simulink model "Model_TranslationEngine64"  (R2022b)
settings: Solver=FixedStepDiscrete  StartTime=0.0  StopTime=5  RelTol=1e-3  EnableMultiTasking=on
InitFcn:
  | % Initialize model
  | ModelSettings=BTConfig.GetModelSettings();
  | 
  | ModelSettings.Validate();
  | 
  | ModelInit;
  | 
  | 
  | % load library data
  | GainLibrary_data;
  | % Load saved values from partition process
  | CapturedConstMask.LoadMapFromFile(bdroot)
StartFcn:
  | % make sure all the simulated RTC requests are found
  | %RTC_SIM_OBJ.ValidateREQs();
undefined symbols (not defined in the file or in its folder): AA, BPLP, Column, NumHFRefBPF, NumHFRefLPF, NumMusicChannels, Row, VolumeMuteConfig
libraries: TuneVar x925, TOP x490, FeaturePath x111, CapturedConstLib x52
(part 34 of 34)

== matlab function Model_TranslationEngine64/ModelPreAmp/DecRate/Medusa5H1/MedusaHoligram/Medusa5H1 Part 3/On/Expand Tail Components/Tail Component EQ/InnerLink/PoolIirTunableWithReset/Translation ==
  data: RawSOS input; NumStages input; PoolNumStages output; PoolCoeffs output; MaxNumStages parameter; VariantUint8 parameter; NumChannels input
  events: trigger input FUNCTION_CALL_EVENT
function [PoolNumStages, PoolCoeffs] = pooliirTranslation(RawSOS, NumStages, MaxNumStages, VariantUint8,  NumChannels)
%#codegen

% Translation from raw SOS for pool SOS

% Some build time sanity size checking before calling the translation
if numel(NumStages.Value) ~= NumChannels
    error('Size of num stages has to match number of input channels')
end

if RawSOS.Size(2) ~= 6
    error ('Coefficient pool matrix must have 6 columns')
end

[PoolNumStages, PoolCoeffs] = poolIirTranslation(RawSOS, NumStages, MaxNumStages, VariantUint8);

% VariantStr = char(VariantUint8);
% switch (VariantStr)
%     case {"Generic","SharcPlusCore"}
%         % These variants order biquad coefficients in a compacted form
%         [PoolNumStages, PoolCoeffs] = pooliirTranslationFcn(RawSOS, NumStages, MaxNumStages);
%     case {"SharcPlusAccelGul","SharcPlusAccelGxp"}
%         % These variants order biquad coefficients for the ADI accelerator
%         [PoolNumStages, PoolCoeffs] = pooliirAccelTranslationFcn(RawSOS, NumStages, MaxNumStages);
%     case{"Hexagon"}
%         % Hexagon specific order for biquad coefficients 
%         [PoolNumStages, PoolCoeffs] = PoolIirHexagonTranslationFcn(RawSOS, NumStages, MaxNumStages);
%     case{"ArmNeonV7V8"}
%         [PoolNumStages, PoolCoeffs] = PoolIirArmNeonV7V8TranslationFcn(RawSOS, NumStages, MaxNumStages);
%     otherwise
%         % This is a build-time error, not a translation error. The
%         % selected build-time variant is not supported for translation
%         error('Invalid implementation type: [%s]', VariantStr);
% end

end

== matlab function Model_TranslationEngine64/NEAR/Near1p1/VolumeMute/VolMuteCh1/Ann1NonEntVncApplied/nonentVNCApplied_subsystem/TuneTOP/Translation ==
  data: Num output; tau input; Fs input; L input; Den output
  events: trigger input FUNCTION_CALL_EVENT
function [Num, Den]  = fcn(tau, Fs, L)

f0 = 1/tau.Value;   % Approximation of cutoff freq from lpf filter time constant

fs_lpf = Fs/L;        % lpf filtter sample rate

% [Num, Den]= butter(1,2*f0/fs_lpf);  % butter() doesn't work with dynamic parameters
[Num, Den] = firstOrderButter(fs_lpf,f0);  % Calculation of lpf filter coefficients

== matlab function Model_TranslationEngine64/ModelPreAmp/DecRate/Medusa5H1/MedusaHoligram/Medusa5H1 Part 2/SPUM Decay Estimate/Decay Estimate/Trivial Translation ==
  data: PSDSmoothFactor output; PSDSmoothCutoff input; FrameRate input
  events: trigger input FUNCTION_CALL_EVENT
function PSDSmoothFactor  = fcn(PSDSmoothCutoff, FrameRate)
% Cutoff is the inverse of time constant in Hz. So this function
% basically converts reciprocal of time constant to first order iir
% filter coefficient.
% Reference: https://bosecorp.sharepoint.com/sites/ASD3/DSPTeam/Shared%20Documents/DSP_Topics/Comparison%20of%20time%20constant%20conversion%20methods.docx
wn = 2 * pi * PSDSmoothCutoff.Value / FrameRate;
PSDSmoothFactor = (1 - sin(wn)) ./ cos(wn);
end

== matlab function Model_TranslationEngine64/ModelPreAmp/DecRate/Medusa5H1/MedusaHoligram/Medusa5H1 Part 2/SPUM Decay Estimate/Decay Estimate/Trivial Translation1 ==
  data: DecaySmoothFactor output; DecaySmoothCutoff input; FrameRate input
  events: trigger input FUNCTION_CALL_EVENT
function DecaySmoothFactor  = fcn(DecaySmoothCutoff, FrameRate)
% Cutoff is the inverse of time constant in Hz. So this function
% basically converts reciprocal of time constant to first order iir
% filter coefficient.
% Reference: https://bosecorp.sharepoint.com/sites/ASD3/DSPTeam/Shared%20Documents/DSP_Topics/Comparison%20of%20time%20constant%20conversion%20methods.docx
wn = 2 * pi * DecaySmoothCutoff.Value / FrameRate;
DecaySmoothFactor = (1 - sin(wn)) ./ cos(wn);
end

== matlab function Model_TranslationEngine64/ModelPreAmp/DecRate/Medusa5H1/MedusaHoligram/Medusa5H1 Part 2/SPUM Decay Estimate/Decay Estimate/Trivial Translation2 ==
  data: FastAttack output; FastAttackCutoff input; SlowAttackCutoff input; FrameRate input; SlowAttack output
  events: trigger input FUNCTION_CALL_EVENT
function [FastAttack, SlowAttack] = fcn(FastAttackCutoff, SlowAttackCutoff, FrameRate)
% Cutoff is the inverse of time constant in Hz. So this function
% basically converts reciprocal of time constant to first order iir
% filter coefficient.
% Reference: https://bosecorp.sharepoint.com/sites/ASD3/DSPTeam/Shared%20Documents/DSP_Topics/Comparison%20of%20time%20constant%20conversion%20methods.docx
if FastAttackCutoff.Value >= SlowAttackCutoff.Value
    wn = 2 * pi * FastAttackCutoff.Value / FrameRate;
    FastAttack = 1 - (1 - sin(wn)) ./ cos(wn);
    wn = 2 * pi * SlowAttackCutoff.Value / FrameRate;
    SlowAttack = 1 - (1 - sin(wn)) ./ cos(wn);
else
    TranslateError('Cutoff frequency of single pole averager for '...
        ,'decay should be less than or equal to that for attack');
    FastAttack = 0;
    SlowAttack = 0;
end

== matlab function Model_TranslationEngine64/ModelPreAmp/DecRate/Medusa5H1/MedusaHoligram/Medusa5H1 Part 2/SPUM Decay Estimate/Decay Estimate/Trivial Translation3 ==
  data: StepIncrement output; StepSize input; FrameRate input; StepDecrement output
  events: trigger input FUNCTION_CALL_EVENT
function [StepIncrement, StepDecrement] = fcn(StepSize, FrameRate)

if StepSize.Value >= 0
    StepIncrement = StepSize.Value/FrameRate;
    StepDecrement = -StepSize.Value/FrameRate;
else
    TranslateError('Step size for slewing should be greater than or equal to zero.');
    StepIncrement = 0;
    StepDecrement = 0;
end

== matlab function Model_TranslationEngine64/ModelPreAmp/DecRate/Medusa5H1/MedusaHoligram/Medusa5H1 Part 2/SPUM Decay Estimate/Decay Estimate/Trivial Translation4 ==
  data: directPathSec input; FrameRate input; DirectPathFramesFs output
  events: trigger input FUNCTION_CALL_EVENT
function DirectPathFramesFs  = fcn(directPathSec, FrameRate)

% Convert delay in seconds to number of full-rate frames
DirectPathFramesFs = round(directPathSec.Value*FrameRate);

end

== matlab function Model_TranslationEngine64/ModelPreAmp/DecRate/Medusa5H1/MedusaHoligram/Medusa5H1 Part 2/Full-Rate FDP/Fdp/FreqDomainProcessing/CalculateAndApplyCoefficients/FullRate/Calculate coefficients/StretchParams/Trivial Translation ==
  data: XpMax output; XpMaxIn input; LokRokMaxScaleFactor output; XpMinIn input; XpMin output; deciXpMaxIn input
  events: trigger input FUNCTION_CALL_EVENT
function [XpMax, LokRokMaxScaleFactor,  XpMin] = fcn(XpMaxIn, XpMinIn, deciXpMaxIn)

XpMax = XpMaxIn.Value;
XpMin = XpMinIn.Value;

if (XpMin < 0) || (XpMin >= 1)
    TranslateError('XpMin must be no less than 0.0, and must be less than 1.0');
end

if (XpMax < 0) || (XpMax >= 1)
    TranslateError('XpMax must be no less than 0.0, and must be less than 1.0');
end

if (XpMax < XpMin)
    TranslateError('XpMin cannot exceed XpMax');
end

% Do not need to check for translation error as this is already done in
% Decimated Rate block.
deciXpMax = deciXpMaxIn.Value; 

% NOTE: The Xp used for detect is the decimated rate Xp while the Xp
% used for the XpMax (in the dynamically created Xp) is the treble Xp.
% All parameters are also treble-specific (different from decimated rate).
% This means the LokRokMaxScaleFactor for treble stretching is calculated
% using the decimated rate XpMax.
if (deciXpMax == 1)
    LokRokMaxScaleFactor = 0;
else
    LokRokMaxScaleFactor = 0.5 * deciXpMax / (1 - deciXpMax);
end

end

== matlab function Model_TranslationEngine64/ModelPreAmp/DecRate/Medusa5H1/MedusaHoligram/Medusa5H1 Part 2/Full-Rate FDP/Fdp/FreqDomainProcessing/CalculateAndApplyCoefficients/FullRate/Calculate coefficients/StretchParams/Trivial Translation3 ==
  data: ESDUpperbounddBIn input; ESDUpperbounddB output; ESDLowerbounddB output; ESDLowerbounddBIn input; ESDStepSize output
  events: trigger input FUNCTION_CALL_EVENT
function [ESDUpperbounddB, ESDLowerbounddB, ESDStepSize]  = ...
                fcn(ESDUpperbounddBIn, ESDLowerbounddBIn)
            
if (ESDUpperbounddBIn.Value >= ESDLowerbounddBIn.Value)
    ESDUpperbounddB = ESDUpperbounddBIn.Value;
    ESDLowerbounddB = ESDLowerbounddBIn.Value;
else    
    TranslateError('Lower threshold for ESD cannot exceed upper threshold for ESD');
    ESDUpperbounddB = 0;
    ESDLowerbounddB = 0;
end

if (ESDUpperbounddBIn.Value == ESDLowerbounddBIn.Value)
    ESDStepSize = 0;
else
    ESDStepSize = 1/abs(ESDUpperbounddBIn.Value - ESDLowerbounddBIn.Value);
end

end

== matlab function Model_TranslationEngine64/ModelPreAmp/DecRate/Medusa5H1/MedusaHoligram/Medusa5H1 Part 4/On/DR Mix Matrix with Hybrid Holigram EQ/IIR/PoolIirTunableWithReset/Translation ==
  data: RawSOS input; NumStages input; PoolNumStages output; PoolCoeffs output; MaxNumStages parameter; VariantUint8 parameter; NumChannels input
  events: trigger input FUNCTION_CALL_EVENT
function [PoolNumStages, PoolCoeffs] = pooliirTranslation(RawSOS, NumStages, MaxNumStages, VariantUint8,  NumChannels)
%#codegen

% Translation from raw SOS for pool SOS

% Some build time sanity size checking before calling the translation
if numel(NumStages.Value) ~= NumChannels
    error('Size of num stages has to match number of input channels')
end

if RawSOS.Size(2) ~= 6
    error ('Coefficient pool matrix must have 6 columns')
end

[PoolNumStages, PoolCoeffs] = poolIirTranslation(RawSOS, NumStages, MaxNumStages, VariantUint8);

% VariantStr = char(VariantUint8);
% switch (VariantStr)
%     case {"Generic","SharcPlusCore"}
%         % These variants order biquad coefficients in a compacted form
%         [PoolNumStages, PoolCoeffs] = pooliirTranslationFcn(RawSOS, NumStages, MaxNumStages);
%     case {"SharcPlusAccelGul","SharcPlusAccelGxp"}
%         % These variants order biquad coefficients for the ADI accelerator
%         [PoolNumStages, PoolCoeffs] = pooliirAccelTranslationFcn(RawSOS, NumStages, MaxNumStages);
%     case{"Hexagon"}
%         % Hexagon specific order for biquad coefficients 
%         [PoolNumStages, PoolCoeffs] = PoolIirHexagonTranslationFcn(RawSOS, NumStages, MaxNumStages);
%     case{"ArmNeonV7V8"}
%         [PoolNumStages, PoolCoeffs] = PoolIirArmNeonV7V8TranslationFcn(RawSOS, NumStages, MaxNumStages);
%     otherwise
%         % This is a build-time error, not a translation error. The
%         % selected build-time variant is not supported for translation
%         error('Invalid implementation type: [%s]', VariantStr);
% end

end

== matlab function Model_TranslationEngine64/ModelPreAmp/DecRate/Medusa5H1/MedusaHoligram/Medusa5H1 Part 3/On/VLS Gains Computation/VLS Gains Drv/Fade Tuning/Backward Downmix Max/Trivial Translation ==
  data: TOP output; BackwardDownmixMax input
  events: trigger input FUNCTION_CALL_EVENT
function TOP  = fcn(BackwardDownmixMax)
%#codegen
% Checks if the parameter satisfies dimensionality requirements
if(numel(BackwardDownmixMax.Value) ~= 1)
   TranslateError('The parameter ''medusa_backward_downmix_max'' must be single dimensional.'); 
end

% Checks if the parameter value follows bound requirements
if((BackwardDownmixMax.Value < 0) || (BackwardDownmixMax.Value > 1))
   TranslateError('The value of ''medusa_backward_downmix_max'' must be between 0 and 1.'); 
end

TOP = BackwardDownmixMax.Value;

end

== matlab function Model_TranslationEngine64/ModelPreAmp/DecRate/Medusa5H1/MedusaHoligram/Medusa5H1 Part 2/Decimated-Rate FDP/Fdp/FreqDomainProcessing/Reverb Extractions/Trivial Translation1 ==
  data: FastPsdSmoothFactor output; FastPsdSmoothCutoff input; SlowPsdSmoothFactor output; SlowPsdSmoothCutoff input; FrameRate input
  events: trigger input FUNCTION_CALL_EVENT
function [FastPsdSmoothFactor, SlowPsdSmoothFactor]  = fcn(FastPsdSmoothCutoff, SlowPsdSmoothCutoff, FrameRate)
% Cutoff is the inverse of time constant in Hz. So this function
% basically converts reciprocal of time constant to first order iir
% filter coefficient.
% Reference: https://bosecorp.sharepoint.com/sites/ASD3/DSPTeam/Shared%20Documents/DSP_Topics/Comparison%20of%20time%20constant%20conversion%20methods.docx

if FastPsdSmoothCutoff.Value >= SlowPsdSmoothCutoff.Value
    wn = 2 * pi * FastPsdSmoothCutoff.Value / FrameRate;
    FastPsdSmoothFactor = (1 - sin(wn)) ./ cos(wn);
    wn = 2 * pi * SlowPsdSmoothCutoff.Value / FrameRate;
    SlowPsdSmoothFactor = (1 - sin(wn)) ./ cos(wn);
else
    TranslateError('Cutoff frequency of single pole averager for smoothing'... 
       ,'fast PSD should be less than or equal to that for smoothing slow PSD.');
    FastPsdSmoothFactor = 0;
    SlowPsdSmoothFactor = 0;
end

== matlab function Model_TranslationEngine64/NEAR/Near1p1/NearBandSplit/HighpassFilter/Translation ==
  data: LRHighPassNumStages output; LRHighPassCoeffs output; crossOverFrequency input; order input; sampleRate input; numChannels input
  events: trigger input FUNCTION_CALL_EVENT
function [LRHighPassNumStages, LRHighPassCoeffs]  = fcn(crossOverFrequency, order, sampleRate, numChannels)
%#codegen
MAX_HPF_ORDER = 10;
MAX_NUM_CHANNELS = 4;
IIR_HIGHPASS = 1;

% Linkwitz-Riley Filters can be construed as the cascade of
% two Butterworth Filters of half the order at the same frequency.
filterOrder = order.Value;
butterOrder = floor((filterOrder+1)/2);
normFrequency = crossOverFrequency.Value/(sampleRate/2);

% High-pass Filters
[halfZ, halfP, halfK] = CalcButterworth(butterOrder,normFrequency,IIR_HIGHPASS);
fullZ = [halfZ halfZ];                         % zeros
fullP = [halfP halfP];                         % poles
fullK = halfK*halfK;                           % gain
sosHighPass = zp2sos(fullZ,fullP,fullK);

% Generate Linkwitz-Riley Pair Coefficients
maxFilterOrder = MAX_HPF_ORDER;
maxNumChannels = MAX_NUM_CHANNELS;
numStages = uint32(size(sosHighPass, 1) * ones(1, maxNumChannels));
maxNumStages = maxFilterOrder * maxNumChannels;

LRHighPassNumStages = uint32(zeros(maxNumChannels,1));
LRHighPassCoeffs = single(zeros((maxNumStages * 4 + maxNumChannels),1));

rawSOSHighPass = repmat(sosHighPass, 4, 1);
[LRHighPassNumStages, LRHighPassCoeffs] = pooliirTranslation(rawSOSHighPass, numStages, maxNumStages, numChannels, maxNumChannels);

end

function [PoolNumStages, PoolCoeffs] = pooliirTranslation(rawSOS, numStages, maxNumStages, numChannels, maxNumChannels)

RawSOS = rawSOS;
NumStages = uint32(numStages);
NumChannels = numChannels;

MaxNumStages = maxNumStages; 
PoolNumStages = uint32(zeros(maxNumChannels,1));
PoolCoeffs = single(zeros(MaxNumStages * 4 + maxNumChannels,1));
ChannelCoeffs = zeros(MaxNumStages * 4 + 1,1);
ChannelSOS = single(zeros(MaxNumStages, 6));
SOSIndex = uint32(0);


for i = 1:NumChannels
    
    ChannelNumStages = NumStages(i);   % Size of current SOS
    assert(ChannelNumStages <= MaxNumStages);
    
    if (ChannelNumStages == 0)
        continue;
    end
    
    ChannelSOS(1:ChannelNumStages,:) = RawSOS(SOSIndex+(1:ChannelNumStages),:);
    SOSIndex = SOSIndex + ChannelNumStages;

    if size(ChannelSOS,2) ~= 6
        TranslateError('SOS matrix must have 6 columns');
    end
    % decompose SOS
   
    ts = 1:4:4*ChannelNumStages;
    ChannelCoeffs(1,1) = prod(ChannelSOS(1:ChannelNumStages,1));        % b0
	
	% Error out for poorly-formed sos coeffs
	if ((ChannelCoeffs(1,1) == 0) && (ChannelNumStages > 1))
		TranslateError('Poorly-formed SOS: zero b0 for multi-stage results in a zero EQ.');
	end
    
    % the remaining coeffs are compacted forms of the biquads
    ChannelCoeffs(1+ts,1) = ChannelSOS(1:ChannelNumStages,6);           % a2
    ChannelCoeffs(2+ts,1) = ChannelSOS(1:ChannelNumStages,5);           % a1
    if( any(ChannelSOS(1:ChannelNumStages,1) == 0 ))
    ChannelCoeffs(3+ts,1) = 0;                 % b2/b0
    ChannelCoeffs(4+ts,1) = 0;                 % b1/b0
    else
    ChannelCoeffs(3+ts,1) = ...
        ChannelSOS(1:ChannelNumStages,3)./ ...
        ChannelSOS(1:ChannelNumStages,1);  % b2/b0
    ChannelCoeffs(4+ts,1) = ...
        ChannelSOS(1:ChannelNumStages,2)./ ...
        ChannelSOS(1:ChannelNumStages,1);  % b1/b0
    end
    
    % length of Cuurent Channel Coeffs
    
    ChannelCoeffsLength = 1+4*ChannelNumStages;
    
    % Offset into coefficient array for the current channel
    offset = uint32((i-1)+4*sum(PoolNumStages(1:i-1)));
    
    % Verify that the SOS does not violate the maximum number of stages
    % allocated for the pool
    PoolNumStages(i) = int32(ChannelNumStages);
    if sum(PoolNumStages) > MaxNumStages
        TranslateError('Too many second order sections');
    end

    % Store the coefficients
    PoolCoeffs(offset+(1:ChannelCoeffsLength)) = single(ChannelCoeffs(1:ChannelCoeffsLength));   
end
end

function [z,p,k] = CalcButterworth(order,frequency,filterType)
MAX_HPF_ORDER = 10;
IIR_HIGHPASS = 1;

    if order > MAX_HPF_ORDER
       order = MAX_HPF_ORDER;
    end
            
    % zeros first
    z = zeros(1,order);
    if filterType == IIR_HIGHPASS
        z(1:order) = ones(1,min(order,MAX_HPF_ORDER));
    elseif filterType == IIR_LOWPASS
        z(1:order) = -1*ones(1,min(order,MAX_HPF_ORDER));
    else
        TranslateError('Filter Type must be high or low');
    end

    p = complex(zeros(1,MAX_HPF_ORDER));
    for n = 1:order
        if n == (order+1)/2 
            sp = -pi*frequency;
        else
            sp_real = pi*frequency*cos(((2*n+order-1)*pi)/(2*order));
            sp_imag = pi*frequency*sin(((2*n+order-1)*pi)/(2*order));
            sp = sp_real + 1i*sp_imag;
        end

        p(n) = (1+sp/2)/(1-sp/2);
    end

    z = z(1:order);
    p = p(1:order);

    if filterType == IIR_HIGHPASS
        k = real(prod((1+p(1:order))/2));
    else 
        k = real(prod((1-p(1:order))/2));
    end
end

% The zp2sos Function stated below supports code generation! 
% Most of the code is scripted refering to the Matlab's zp2sos.m and
% https://searchcode.com/codesearch/view/9505959/ 
% Integration of two codes was majorily required due to cplxreal function 
% which is no more supported in Matlab Scripts. 
function [sos,g] = zp2sos(z,p,g)
    if nargin < 3
        g = 1; 
    end
    if nargin < 2
        p = []; 
    end

    % Sort the numbers z into complex-conjugate-valued and real-valued elements.
    % The positive imaginary complex numbers of each complex conjugate pair 
    % are returned in zc and the real numbers are returned in zr.

    % pair up the conjugate poles and zeros using cplxpair
    z = cplxpair(z);
    p = cplxpair(p);

    % Get the number of poles and zeros
    lz = length(z);
    lp = length(p);

    ind = find(abs(imag(p)) > 0);
    p_conj = p(ind);   % poles that have conjugate pairs

    coder.varsize('ind_complement');
    B = p_conj(imag(p_conj) >= 0);
    ind_complement = 1:lp;
    if ~isempty(ind)
        ind_complement(ind) = [];
    end
    p_real = p(ind_complement);    % poles that are real

    % break up conjugate pairs and real zeros
    ind = find(abs(imag(z)) > 0);
    z_conj = z(ind);   % zeros that have conjugate pairs
    C = z_conj(imag(z_conj) >= 0);
    ind_complement = 1:lz;
    if ~isempty(ind)
       ind_complement(ind) = [];
    end
    z_real = z(ind_complement);

    zr = z_real; % zeroes that are real
    pr = p_real ;% poles that are real
    pc = B; % positive conjugate poles
    zc = C ; % positive conjugate zeros

    % zc,zr,pc,pr found

    nzc = length(zc);
    npc = length(pc);

    nzr = length(zr);
    npr = length(pr);

    % Pair up real zeros:
    if nzr
        if mod(nzr,2)==1
            zr_temp = [zr;0]; 
            nzr = nzr+1; 
        else
            zr_temp = zr;
        end
        nzrsec = nzr/2;
        zrms = real(-zr_temp(1:2:nzr-1) - zr_temp(2:2:nzr));
        zrp = real(zr_temp(1:2:nzr-1) .* zr_temp(2:2:nzr));
    else
        nzrsec = 0;
        zrms = 0; 
        zrp = 0;
    end

    % Pair up real poles:
    if npr
        if mod(npr,2) == 1
            pr_temp = [pr;0]; 
            npr = npr+1; 
        else
            pr_temp = pr;
        end
        nprsec = npr/2;
        prms = real(-pr_temp(1:2:npr-1) - pr_temp(2:2:npr));
        prp = real(pr_temp(1:2:npr-1) .* pr_temp(2:2:npr));
    else
        nprsec = 0;
        prp = 0;
        prms = 0;
    end

    nsecs = max(ceil(lz/2), ceil(lp/2));

    % Convert complex zeros and poles to real 2nd-order section form:
    zcm2r = -2*real(zc);
    zca2 = abs(zc) .^ 2;
    pcm2r = -2 * real(pc);
    pca2 = abs(pc) .^ 2;

    sos = zeros(nsecs, 6);
    sos(:,1) = ones(nsecs, 1); % all 2nd-order polynomials are monic
    sos(end,1) = g*sos(end, 1);
    sos(:,4) = ones(nsecs, 1); 

    nzrl = nzc + nzrsec; % index of last real zero section
    nprl = npc + nprsec; % index of last real pole section

    for i = 1:nsecs

        if i <= nzc % lay down a complex zero pair:
            sos(i,2:3) = [zcm2r(i) zca2(i)];
            sos(end,2:3) = g*sos(end,2:3);
        elseif i <= nzrl % lay down a pair of real zeros:
            sos(i,2:3) = [zrms(i-nzc) zrp(i-nzc)];
            sos(end,2:3) = g*sos(end,2:3);
        end  

        if i <= npc % lay down a complex pole pair:
            sos(i,5:6) = [pcm2r(i) pca2(i)];
        elseif i <= nprl % lay down a pair of real poles:
            sos(i,5:6) = [prms(i-npc) prp(i-npc)];
        end  
    end        
end

== matlab function Model_TranslationEngine64/ModelPreAmp/DecRate/Medusa5H1/MedusaHoligram/Medusa5H1 Part 2/Decimated-Rate FDP/Fdp/FreqDomainProcessing/Reverb Extractions/Trivial Translation3 ==
  data: DirectPathDec output; DirectPathSec input; FrameRate input; FrameSize input
  events: trigger input FUNCTION_CALL_EVENT
function DirectPathDec  = fcn(DirectPathSec, FrameRate, FrameSize)

DirectPathDec = round(DirectPathSec.Value*FrameRate)*FrameSize;

end

== matlab function Model_TranslationEngine64/ModelPreAmp/DecRate/Medusa5H1/MedusaHoligram/Medusa5H1 Part 2/Decimated-Rate FDP/Fdp/FreqDomainProcessing/Reverb Extractions/Trivial Translation4 ==
  data: LsSmoothFactor output; LsSmoothCutoff input; FrameRate input
  events: trigger input FUNCTION_CALL_EVENT
function LsSmoothFactor  = fcn(LsSmoothCutoff, FrameRate)

% Cutoff is the inverse of time constant in Hz. So this function
% basically converts reciprocal of time constant to first order iir
% filter coefficient.
% Reference: https://bosecorp.sharepoint.com/sites/ASD3/DSPTeam/Shared%20Documents/DSP_Topics/Comparison%20of%20time%20constant%20conversion%20methods.docx
wn = 2 * pi * LsSmoothCutoff.Value / FrameRate;
LsSmoothFactor = (1 - sin(wn)) ./ cos(wn);

end

== matlab function Model_TranslationEngine64/ModelPreAmp/DecRate/Medusa5H1/MedusaHoligram/Medusa5H1 Part 3/On/VLS Gains Computation/VLS Gains Drv/Fade Tuning/Backward Downmix Threshold/Trivial Translation ==
  data: TOP output; BackwardDownmixThreshold input
  events: trigger input FUNCTION_CALL_EVENT
function TOP  = fcn(BackwardDownmixThreshold)
%#codegen
% Checks if the parameter satisfies dimensionality requirements
if(numel(BackwardDownmixThreshold.Value) ~= 1)
   TranslateError('The parameter ''medusa_backward_downmix_threshold'' must be single dimensional.'); 
end

% Checks if the parameter value follows bound requirements
if((BackwardDownmixThreshold.Value < 0) || (BackwardDownmixThreshold.Value > 1))
   TranslateError('The value of ''medusa_backward_downmix_threshold'' must be between 0 and 1.'); 
end

TOP = BackwardDownmixThreshold.Value;

end

== matlab function Model_TranslationEngine64/ModelPreAmp/DecRate/Medusa5H1/MedusaHoligram/Medusa5H1 Part 3/On/VLS Gains Computation/VLS Gains Drv/Fade Tuning/Downmix Weights/Trivial Translation ==
  data: TOP output; downmix_wts input; configStruct parameter
  events: trigger input FUNCTION_CALL_EVENT
function TOP  = fcn(downmix_wts, configStruct)
%#codegen

% Checks if the parameter satisfies dimensionality requirements
if(downmix_wts.Size(1) ~= configStruct.numGains)
    TranslateError('The parameter ''VLS_downmix'' must be a %d element vector.', configStruct.numGains);
end

% Checks if the parameter values follow bound requirements
checkValues = (downmix_wts.Value < 0);
if(sum(sum(checkValues)))          % Results in 0 if all values in the matrix respect the bound requirements
    TranslateError('The weights in ''VLS_downmix'' must be greater than or equal to 0.');
end

TOP = downmix_wts.Value;

end

== matlab function Model_TranslationEngine64/ModelPreAmp/DecRate/Medusa5H1/MedusaHoligram/Medusa5H1 Part 2/Full-Rate FDP/Fdp/FreqDomainProcessing/Reverb Extractions/Trivial Translation1 ==
  data: FastPsdSmoothFactor output; FastPsdSmoothCutoff input; SlowPsdSmoothFactor output; SlowPsdSmoothCutoff input; FrameRate input
  events: trigger input FUNCTION_CALL_EVENT
function [FastPsdSmoothFactor, SlowPsdSmoothFactor]  = fcn(FastPsdSmoothCutoff, SlowPsdSmoothCutoff, FrameRate)
% Cutoff is the inverse of time constant in Hz. So this function
% basically converts reciprocal of time constant to first order iir
% filter coefficient.
% Reference: https://bosecorp.sharepoint.com/sites/ASD3/DSPTeam/Shared%20Documents/DSP_Topics/Comparison%20of%20time%20constant%20conversion%20methods.docx

if FastPsdSmoothCutoff.Value >= SlowPsdSmoothCutoff.Value
    wn = 2 * pi * FastPsdSmoothCutoff.Value / FrameRate;
    FastPsdSmoothFactor = (1 - sin(wn)) ./ cos(wn);
    wn = 2 * pi * SlowPsdSmoothCutoff.Value / FrameRate;
    SlowPsdSmoothFactor = (1 - sin(wn)) ./ cos(wn);
else
    TranslateError('Cutoff frequency of single pole averager for smoothing'... 
       ,'fast PSD should be less than or equal to that for smoothing slow PSD.');
    FastPsdSmoothFactor = 0;
    SlowPsdSmoothFactor = 0;
end

== matlab function Model_TranslationEngine64/ModelPreAmp/DecRate/Medusa5H1/MedusaHoligram/Medusa5H1 Part 2/Full-Rate FDP/Fdp/FreqDomainProcessing/Reverb Extractions/Trivial Translation3 ==
  data: DirectPathDec output; DirectPathSec input; FrameRate input; FrameSize input
  events: trigger input FUNCTION_CALL_EVENT
function DirectPathDec  = fcn(DirectPathSec, FrameRate, FrameSize)

DirectPathDec = round(DirectPathSec.Value*FrameRate)*FrameSize;

end

== matlab function Model_TranslationEngine64/ModelPreAmp/DecRate/Medusa5H1/MedusaHoligram/Medusa5H1 Part 2/Full-Rate FDP/Fdp/FreqDomainProcessing/Reverb Extractions/Trivial Translation4 ==
  data: LsSmoothFactor output; LsSmoothCutoff input; FrameRate input
  events: trigger input FUNCTION_CALL_EVENT
function LsSmoothFactor  = fcn(LsSmoothCutoff, FrameRate)

% Cutoff is the inverse of time constant in Hz. So this function
% basically converts reciprocal of time constant to first order iir
% filter coefficient.
% Reference: https://bosecorp.sharepoint.com/sites/ASD3/DSPTeam/Shared%20Documents/DSP_Topics/Comparison%20of%20time%20constant%20conversion%20methods.docx
wn = 2 * pi * LsSmoothCutoff.Value / FrameRate;
LsSmoothFactor = (1 - sin(wn)) ./ cos(wn);

end

== matlab function Model_TranslationEngine64/ModelPreAmp/DecRate/Medusa5H1/MedusaHoligram/Medusa5H1 Part 3/On/VLS Gains Computation/VLS Gains Drv/Fade Tuning/Forward Downmix Threshold/Trivial Translation ==
  data: TOP output; ForwardDownmixThreshold input
  events: trigger input FUNCTION_CALL_EVENT
function TOP  = fcn(ForwardDownmixThreshold)
%#codegen
% Checks if the parameter satisfies dimensionality requirements
if(numel(ForwardDownmixThreshold.Value) ~= 1)
   TranslateError('The parameter ''medusa_forward_downmix_threshold'' must be single dimensional.'); 
end

% Checks if the parameter value follows bound requirements
if((ForwardDownmixThreshold.Value < 0) || (ForwardDownmixThreshold.Value > 1))
   TranslateError('The value of ''medusa_forward_downmix_threshold'' must be between 0 and 1.'); 
end

TOP = ForwardDownmixThreshold.Value;

end

== matlab function Model_TranslationEngine64/ModelPreAmp/DecRate/Medusa5H1/MedusaHoligram/Medusa5H1 Part 3/On/VLS Gains Computation/VLS Gains Drv/Fade Tuning/Foward Downmix Max/Trivial Translation ==
  data: TOP output; ForwardDownmixMax input
  events: trigger input FUNCTION_CALL_EVENT
function TOP  = fcn(ForwardDownmixMax)
%#codegen
% Checks if the parameter satisfies dimensionality requirements
if(numel(ForwardDownmixMax.Value) ~= 1)
   TranslateError('The parameter ''medusa_forward_downmix_max'' must be single dimensional.'); 
end

% Checks if the parameter value follows bound requirements
if((ForwardDownmixMax.Value < 0) || (ForwardDownmixMax.Value > 1))
   TranslateError('The value of ''medusa_forward_downmix_max'' must be between 0 and 1.'); 
end

TOP = ForwardDownmixMax.Value;

end

== matlab function Model_TranslationEngine64/ModelPreAmp/DecRate/Medusa5H1/MedusaHoligram/Medusa5H1 Part 3/On/VLS Gains Computation/VLS Gains Pax/Fade Tuning/Backward Downmix Max/Trivial Translation ==
  data: TOP output; BackwardDownmixMax input
  events: trigger input FUNCTION_CALL_EVENT
function TOP  = fcn(BackwardDownmixMax)
%#codegen
% Checks if the parameter satisfies dimensionality requirements
if(numel(BackwardDownmixMax.Value) ~= 1)
   TranslateError('The parameter ''medusa_backward_downmix_max'' must be single dimensional.'); 
end

% Checks if the parameter value follows bound requirements
if((BackwardDownmixMax.Value < 0) || (BackwardDownmixMax.Value > 1))
   TranslateError('The value of ''medusa_backward_downmix_max'' must be between 0 and 1.'); 
end

TOP = BackwardDownmixMax.Value;

end

== matlab function Model_TranslationEngine64/ModelPreAmp/DecRate/Medusa5H1/MedusaHoligram/Medusa5H1 Part 3/On/VLS Gains Computation/VLS Gains Pax/Fade Tuning/Backward Downmix Threshold/Trivial Translation ==
  data: TOP output; BackwardDownmixThreshold input
  events: trigger input FUNCTION_CALL_EVENT
function TOP  = fcn(BackwardDownmixThreshold)
%#codegen
% Checks if the parameter satisfies dimensionality requirements
if(numel(BackwardDownmixThreshold.Value) ~= 1)
   TranslateError('The parameter ''medusa_backward_downmix_threshold'' must be single dimensional.'); 
end

% Checks if the parameter value follows bound requirements
if((BackwardDownmixThreshold.Value < 0) || (BackwardDownmixThreshold.Value > 1))
   TranslateError('The value of ''medusa_backward_downmix_threshold'' must be between 0 and 1.'); 
end

TOP = BackwardDownmixThreshold.Value;

end

== matlab function Model_TranslationEngine64/ModelPreAmp/DecRate/Medusa5H1/MedusaHoligram/Medusa5H1 Part 3/On/VLS Gains Computation/VLS Gains Pax/Fade Tuning/Downmix Weights/Trivial Translation ==
  data: TOP output; downmix_wts input; configStruct parameter
  events: trigger input FUNCTION_CALL_EVENT
function TOP  = fcn(downmix_wts, configStruct)
%#codegen

% Checks if the parameter satisfies dimensionality requirements
if(downmix_wts.Size(1) ~= configStruct.numGains)
    TranslateError('The parameter ''VLS_downmix'' must be a %d element vector.', configStruct.numGains);
end

% Checks if the parameter values follow bound requirements
checkValues = (downmix_wts.Value < 0);
if(sum(sum(checkValues)))          % Results in 0 if all values in the matrix respect the bound requirements
    TranslateError('The weights in ''VLS_downmix'' must be greater than or equal to 0.');
end

TOP = downmix_wts.Value;

end

== matlab function Model_TranslationEngine64/ModelPreAmp/DecRate/Medusa5H1/MedusaHoligram/Medusa5H1 Part 3/On/VLS Gains Computation/VLS Gains Drv/SLC Tuning/Detent Level/Trivial Translation ==
  data: TOP output; detentGain input; configStruct parameter
  events: trigger input FUNCTION_CALL_EVENT
function TOP  = fcn(detentGain, configStruct)
%#codegen

% Checks if the parameter satisfies dimensionality requirements
if(detentGain.Size(1) ~= configStruct.numGains)
    TranslateError('The parameter ''VLS_gains_detent'' must be a %d element vector.', configStruct.numGains);
end

% Checks if the parameter values follow bound requirements
checkValues = (detentGain.Value < 0);    
if(sum(sum(checkValues)))       % Results in 0 if all values in the matrix respect the bound requirements
    TranslateError('The weights in ''VLS_gains_detent'' must be greater than or equal to 0.');
end

TOP = detentGain.Value;

end
